simulink model "veh_mdl_demo_v14"  (Simulink 7.0)
settings: Solver=ode3  StartTime=0.0  StopTime=100  FixedStep=0.001  RelTol=1e-3
PreLoadFcn:
  | eng_mdl_demo_v14_setup
InitFcn:
  | eng_mdl_demo_v14_setup
undefined symbols (not defined in the file or in its folder): notex
libraries: ni_annotations_lib x1, hil14_mdl_lib x1
CloseFcn:
  | eng_mdl_demo_v14_close
settings Model: Creator=Eric Bradley  LastModifiedBy=Eric Bradley
settings OptimizationCC: SimCompilerOptimization=On
settings DebuggingCC: InheritedTsInSrcMsg=none  ParameterPrecisionLossMsg=none
settings RTWCC: SystemTargetFile=NIVeriStand.tlc  TemplateMakefile=NIVeriStand_vc.tmf  Description=NI VeriStand Real-Time Target for Release 2007b or later  ProcessScript=NIVeriStand_make_rtw_hook
settings STFCustomTargetCC: GenFloatMathFcnCalls=ANSI_C  MatFileLogging=on  SystemTargetFile=NIVeriStand.tlc
settings CustomProperty: Value=on
settings EnumStrPairs: String=Default

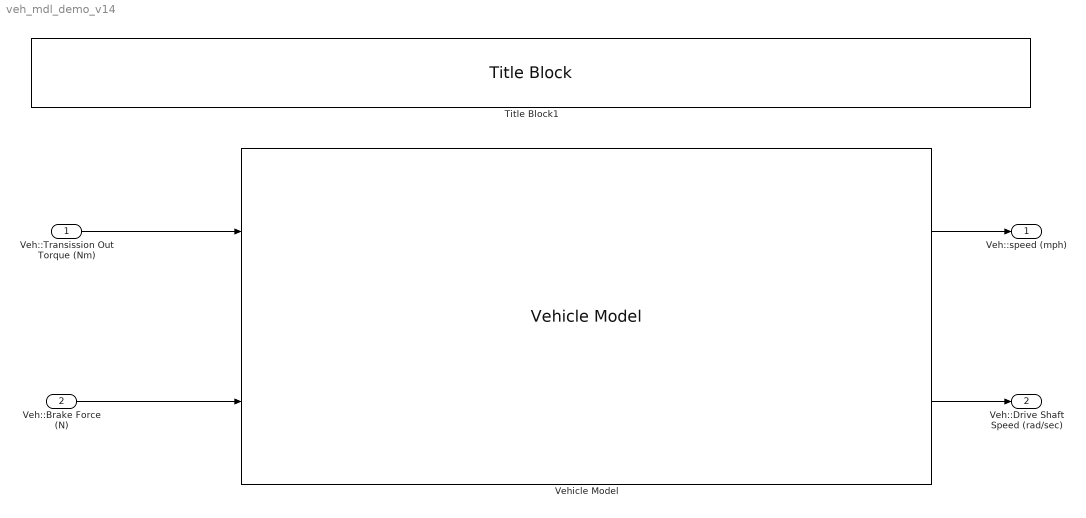
== system veh_mdl_demo_v14 ==
  Veh::Transission Out Torque (Nm) : Inport  OutDataType=sfix(16)  OutScaling=2^0
  Veh::Brake Force (N) : Inport  Port=2  OutDataType=sfix(16)  OutScaling=2^0
  Title Block1 : ni_annotations_lib/Title Block  SystemSampleTime=-1  tx_title=notex(get_param(gcs,'Name'))
  Vehicle Model : hil14_mdl_lib/Vehicle Model  SystemSampleTime=-1  iname='veh.jpg'  scale=0.5
  Veh::speed (mph) : Outport  OutDataType=sfix(16)  OutScaling=2^0
  Veh::Drive Shaft Speed (rad/sec) : Outport  Port=2  OutDataType=sfix(16)  OutScaling=2^0
  wires:
  Vehicle Model/1 -> Veh::speed (mph)/1
  Vehicle Model/2 -> Veh::Drive Shaft Speed (rad/sec)/1
  Veh::Transission Out Torque (Nm)/1 -> Vehicle Model/1
  Veh::Brake Force (N)/1 -> Vehicle Model/2
